simulink model "part_b"  (R2017b)
settings: Solver=VariableStepAuto  StartTime=0.0  StopTime=10.0  RelTol=1e-3
values from neighbouring files (symbols this model uses):
  a = [0 1;-1 -0.7]    [P2a.m]    (also in P2b.m; P2c.m)
  b = [0;1]    [P2a.m]    (also in P2b.m; P2c.m)
  c = [1 0;0 0]    [P2a.m]    (also in P2b.m; P2c.m = [1 0)
undefined symbols (not defined in the file or in its folder): K, L
settings Model: Creator=Soutrik  LastModifiedBy=Soutrik

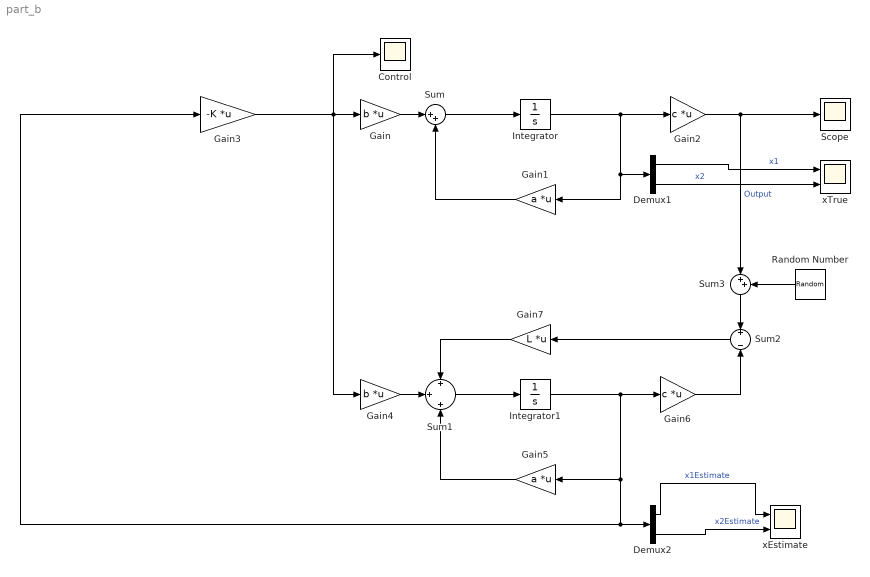
== system part_b ==
  Control : Scope
  Demux1 : Demux  Outputs=2
  Demux2 : Demux  Outputs=2
  Gain : Gain  Gain=b  Multiplication=Matrix(K*u)
  Gain1 : Gain  Gain=a  Multiplication=Matrix(K*u)
  Gain2 : Gain  Gain=c  Multiplication=Matrix(K*u)
  Gain3 : Gain  Gain=-K  Multiplication=Matrix(K*u)
  Gain4 : Gain  Gain=b  Multiplication=Matrix(K*u)
  Gain5 : Gain  Gain=a  Multiplication=Matrix(K*u)
  Gain6 : Gain  Gain=c  Multiplication=Matrix(K*u)
  Gain7 : Gain  Gain=L  Multiplication=Matrix(K*u)
  Integrator : Integrator  InitialCondition=[1 0]
  Integrator1 : Integrator  InitialCondition=[1 0]
  Random Number : RandomNumber  Variance=[0.1,0.1]  Seed=[1 2]  SampleTime=0.01
  Scope : Scope
  Sum : Sum  Inputs=|++
  Sum1 : Sum  Inputs=+|+|+
  Sum2 : Sum  Inputs=+||-
  Sum3 : Sum  Inputs=|++
  xEstimate : Scope  NumInputPorts=2
  xTrue : Scope  NumInputPorts=2
  wires:
  Integrator/1 -> Gain1/1, Demux1/1, Gain2/1
  Gain4/1 -> Sum1/2
  Random Number/1 -> Sum3/2
  Demux2/2 -> xEstimate/2  "x2Estimate"
  Sum3/1 -> Sum2/1
  Demux2/1 -> xEstimate/1  "x1Estimate"
  Gain7/1 -> Sum1/1
  Sum2/1 -> Gain7/1
  Gain5/1 -> Sum1/3
  Demux1/2 -> xTrue/2  "x2"
  Sum1/1 -> Integrator1/1
  Demux1/1 -> xTrue/1  "x1"
  Sum/1 -> Integrator/1
  Gain6/1 -> Sum2/2
  Gain3/1 -> Gain4/1, Gain/1, Control/1
  Gain1/1 -> Sum/2
  Gain2/1 -> Scope/1, Sum3/1  "Output"
  Gain/1 -> Sum/1
  Integrator1/1 -> Gain5/1, Gain3/1, Demux2/1, Gain6/1
